simulink model "PWM_Vel"  (R2023b)
settings: Solver=VariableStepAuto  StartTime=0.0  StopTime=10.0  RelTol=1e-3
settings Model: Creator=Daniel  LastModifiedBy=Daniel

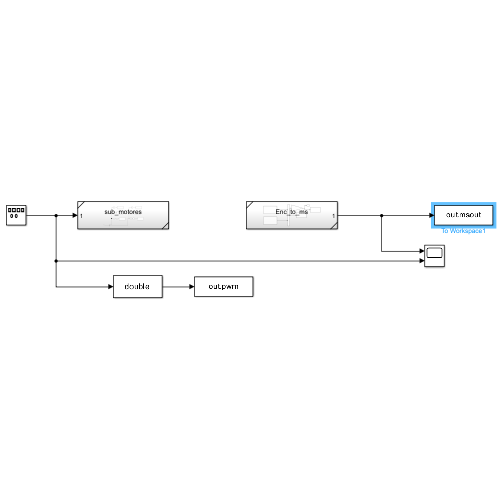
[thumbnail: Simulink's stored preview of the top-level diagram]
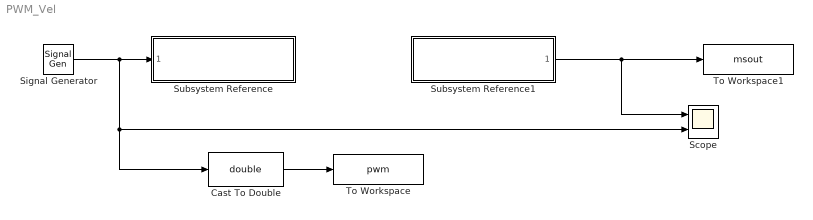
== system PWM_Vel ==
  Cast To Double : DataTypeConversion  OutDataTypeStr=double  SaturateOnIntegerOverflow=off  RndMeth=Floor
  Scope : Scope  NumInputPorts=2
  Signal Generator : SignalGenerator  WaveForm=square  Amplitude=240  Frequency=0.5
  Subsystem Reference : Subsystem  ReferencedSubsystem=sub_motores
  Subsystem Reference1 : Subsystem  ReferencedSubsystem=Enc_to_ms
  To Workspace : ToWorkspace  VariableName=pwm  SaveFormat=Timeseries  SampleTime=-1
  To Workspace1 : ToWorkspace  VariableName=msout  SaveFormat=Timeseries  SampleTime=-1
  wires:
  Signal Generator/1 -> Cast To Double/1, Scope/2, Subsystem Reference/1
  Subsystem Reference1/1 -> Scope/1, To Workspace1/1
  Cast To Double/1 -> To Workspace/1
